simulink model "today5Forsiruschie"  (R2016a)
settings: Solver=VariableStepAuto  StartTime=0.0  StopTime=0.15  RelTol=1e-3
settings Model: Creator=Ivan Varabei  LastModifiedBy=Ivan Varabei

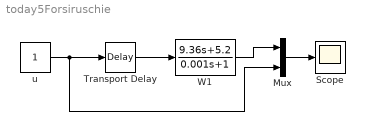
== system today5Forsiruschie ==
  Mux : Mux  Inputs=2
  Scope : Scope
  Transport Delay : TransportDelay  DelayTime=0.1
  "W1 " : TransferFcn  Numerator=[9.36 5.2]  Denominator=[0.001 1]
  u : Constant
  wires:
  Transport Delay/1 -> "W1 "/1
  u/1 -> Mux/2, Transport Delay/1
  Mux/1 -> Scope/1
  "W1 "/1 -> Mux/1
